simulink model "ctrl_PF"  (R2022b)
settings: Solver=FixedStepAuto  StartTime=0.0  StopTime=Tf  FixedStep=0.05  RelTol=1e-3
StopFcn:
  | save('testdata')
values from neighbouring files (symbols this model uses):
  Ba_0 = [0 0 0 0 0 0]    [run.m]    (also in testdata.mat)
  Bb = 4418825.3321    [testdata.mat]
  Bv_0 = [-5.14444 0 0 0 0 0]    [run.m]    (also in testdata.mat)
  Bx_0 = [-Cp(1,1) -Cp(2,1) Cp(3,1) 0 0 -pi]    [run.m]    (also in testdata.mat = [7.34788079488e-14 -400 -100 0 0 -3.14159265359])
  Cp = [x;y;z]    [run.m]    (also in testdata.mat = [-7.34788079488e-14 400 -100 -24.1026674607 399.273166418 -1)
  Cp_prime = Cp*Diff    [run.m]    (also in testdata.mat = [-4.77232815721 -0.143913049279 0 -4.75515990164 -0.42831409)
  d = 50    [run.m]    (also in testdata.mat)
  dA_BP1 = [0.00388591051125 0.00354364911083 0.00553040741788 0.00502167988714 0.0078585088908 0.00748424955325 0.0119232766011 0.0109054787122 0.0168329706434 0.016985509009 0.0156802934897 0.014556760782 ... (616 elements, 616x1)]    [testdata.mat]
  dA_BP2 = [0.00388594063171 0.00354357191533 0.00553040491113 0.00502170939051 0.00785855989083 0.00748435285791 0.0119232653011 0.0109054419481 0.0168329955973 0.0169854794658 0.015680230324 0.0145567225609 ... (616 elements, 616x1)]    [testdata.mat]
  dA_Hull = [0.896301676511 0.898896720864 0.884294141897 0.886832830172 0.870887902011 0.873360353662 0.856223658523 0.858613244346 0.840314828191 0.842595287849 0.823129385532 0.8253007603 ... (2914 elements, 2914x1)]    [testdata.mat]
  dA_PH = [0.00917454029683 0.00917454029683 0.00646521761836 0.00644666811643 0.011728531678 0.0107683420972 0.0165186720105 0.0100399866209 0.0121147162203 0.00917369783051 0.00917369783051 0.00646462373197 ... (550 elements, 550x1)]    [testdata.mat]
  dA_Sail = [0.08073747293 0.0655437895785 0.0678199581962 0.211496702297 0.185444652254 0.10949647106 0.0763960001413 0.0735864235671 0.0440728222699 0.281106392154 0.32735958292 0.104041938486 ... (564 elements, 564x1)]    [testdata.mat]
  dA_SProot = [0.0225345452169 0.0247277274893 0.0225345452169 0.0480467976325 0.0166447079844 0.0410754287554 0.0247277274893 0.0480467976325 0.0468898715351 0.0839833312794 0.0166447079844 0.0255016718 ... (904 elements, 904x1)]    [testdata.mat]
  dA_X1a = [0.0149621011817 0.0166706156701 0.0341149781095 0.0355915100668 0.0512235531199 0.0489176133683 0.0604458424392 0.0503279152264 0.0577124835488 0.0401555322121 0.044833653096 0.0251568218541 ... (200 elements, 200x1)]    [testdata.mat]
  dA_X1b = [0.0149621011817 0.0166706156701 0.0341149781095 0.0355915100668 0.0512235531199 0.0489176133683 0.0604458424392 0.0503279152264 0.0577124835488 0.0401555322121 0.044833653096 0.0251568218541 ... (200 elements, 200x1)]    [testdata.mat]
  dA_X2a = [0.0149620639393 0.0166705502855 0.0341150948266 0.0355913495849 0.051223110376 0.0489180393921 0.0604458270347 0.0503275686692 0.0577128112225 0.0401556683139 0.0448334591683 0.0251566482124 ... (200 elements, 200x1)]    [testdata.mat]
  dA_X2b = [0.0149620639393 0.0166705502855 0.0341150948266 0.0355913495849 0.051223110376 0.0489180393921 0.0604458270347 0.0503275686692 0.0577128112225 0.0401556683139 0.0448334591683 0.0251566482124 ... (200 elements, 200x1)]    [testdata.mat]
  dA_X3a = [0.0149621011817 0.0166706156701 0.0341149781095 0.0355915100668 0.0512235531199 0.0489176133683 0.0604458424392 0.0503279152264 0.0577124835488 0.0401555322121 0.044833653096 0.0251568218541 ... (200 elements, 200x1)]    [testdata.mat]
  dA_X3b = [0.0149621011817 0.0166706156701 0.0341149781095 0.0355915100668 0.0512235531199 0.0489176133683 0.0604458424392 0.0503279152264 0.0577124835488 0.0401555322121 0.044833653096 0.0251568218541 ... (200 elements, 200x1)]    [testdata.mat]
  dA_X4a = [0.0149621011817 0.0166706156701 0.0341149781095 0.0355915100668 0.0512235531199 0.0489176133683 0.0604458424392 0.0503279152264 0.0577124835488 0.0401555322121 0.044833653096 0.0251568218541 ... (200 elements, 200x1)]    [testdata.mat]
  dA_X4b = [0.0149621011817 0.0166706156701 0.0341149781095 0.0355915100668 0.0512235531199 0.0489176133683 0.0604458424392 0.0503279152264 0.0577124835488 0.0401555322121 0.044833653096 0.0251568218541 ... (200 elements, 200x1)]    [testdata.mat]
  Ixx = 52300000    [testdata.mat]
  Ixy = 0    [testdata.mat]
  Ixz = 0    [testdata.mat]
  Iyy = 1375000000    [testdata.mat]
  Iyz = 0    [testdata.mat]
  Izz = 1367000000    [testdata.mat]
  Ky = 1    [run.m]    (also in testdata.mat)
  Mb = 4418825.3321    [testdata.mat]
  n_BP1 = [-0.7747315 -0.03638153 -0.4095958 0 -0.1221389 0 -0.01670914 0 0.005209626 0 0.03404154 0 ... (1848 elements, 616x3)]    [testdata.mat]
  n_BP2 = [-0.774731517 -0.0363815315 -0.409595788 0 -0.122138903 0 -0.0167091396 0 0.00520962616 0 0.0340415388 0 ... (1848 elements, 616x3)]    [testdata.mat]
  n_Hull = [-3.334458e-05 -1.700098e-14 -3.354233e-05 -1.686235e-14 -3.289162e-05 -1.685701e-14 -3.291391e-05 -1.698144e-14 -3.338145e-05 -1.688959e-14 -3.29289e-05 -1.682536e-14 ... (8742 elements, 2914x3)]    [testdata.mat]
  n_PH = [0 0 0.01711651 0.01711627 0.2676807 0.2676804 0.7675173 0.7675174 0.9857236 0 0 0.01711456 ... (1650 elements, 550x3)]    [testdata.mat]
  n_Sail = [-0.05126832 -0.05168081 -0.0485872 -0.03288998 -0.03203588 -0.04435105 -0.04335441 -0.04419429 -0.05169604 0.01094904 0.01649325 -0.03825178 ... (1692 elements, 564x3)]    [testdata.mat]
  n_SProot = [-0.7837688 -0.7969784 -0.7837688 -0.79448 -0.280412 -0.3378876 -0.7969784 -0.79448 -0.7910827 -0.3483897 -0.280412 -0.2790298 ... (2712 elements, 904x3)]    [testdata.mat]
  n_X2a = [-0.283297986 -0.283136904 -0.283195704 -0.28313759 -0.2831586 -0.283137113 -0.28313911 -0.283136606 -0.283121586 -0.283136815 -0.283108413 -0.283138901 ... (600 elements, 200x3)]    [testdata.mat]
  n_X2b = [-0.283297986 -0.283136904 -0.283195704 -0.28313759 -0.2831586 -0.283137113 -0.28313911 -0.283136606 -0.283121586 -0.283136815 -0.283108413 -0.283138901 ... (600 elements, 200x3)]    [testdata.mat]
  n_X3a = [-0.283298 -0.2831369 -0.2831957 -0.2831376 -0.2831586 -0.2831371 -0.2831391 -0.2831366 -0.2831216 -0.2831368 -0.2831084 -0.2831389 ... (600 elements, 200x3)]    [testdata.mat]
  n_X4a = [-0.283298 -0.2831369 -0.2831957 -0.2831376 -0.2831586 -0.2831371 -0.2831391 -0.2831366 -0.2831216 -0.2831368 -0.2831084 -0.2831389 ... (600 elements, 200x3)]    [testdata.mat]
  n_X4b = [-0.283298 -0.2831369 -0.2831957 -0.2831376 -0.2831586 -0.2831371 -0.2831391 -0.2831366 -0.2831216 -0.2831368 -0.2831084 -0.2831389 ... (600 elements, 200x3)]    [testdata.mat]
  nt_BP1 = 616    [testdata.mat]
  nt_BP2 = 616    [testdata.mat]
  nt_Hull = 2914    [testdata.mat]
  nt_PH = 550    [testdata.mat]
  nt_Sail = 564    [testdata.mat]
  nt_SProot = 904    [testdata.mat]
  nt_X1a = 200    [testdata.mat]
  nt_X1b = 200    [testdata.mat]
  nt_X2a = 200    [testdata.mat]
  nt_X2b = 200    [testdata.mat]
  nt_X3a = 200    [testdata.mat]
  nt_X3b = 200    [testdata.mat]
  nt_X4a = 200    [testdata.mat]
  nt_X4b = 200    [testdata.mat]
  Seastate = 0    [run.m]    (also in testdata.mat)
  Tf = 500    [run.m]    (also in testdata.mat)
  v_ref = Bv_0(1)    [run.m]    (also in testdata.mat = -5.14444)
  vt1_BP1 = [-11.0524049722 -10.9924120522 -10.9924120522 -10.8819663922 -10.8819663922 -10.7297166322 -10.7297166322 -10.5070632922 -10.5070632922 -10.1807245522 -10.1807245522 -9.8815181122 ... (1848 elements, 616x3)]    [testdata.mat]
  vt1_BP2 = [-11.0524048318 -10.9924111396 -10.9924111396 -10.8819658306 -10.8819658306 -10.7297157898 -10.7297157898 -10.5070637134 -10.5070637134 -10.1807238502 -10.1807238502 -9.8815188844 ... (1848 elements, 616x3)]    [testdata.mat]
  vt1_Hull = [3.5122487678 3.7304022878 5.2621803278 5.4863499878 6.9866994878 7.2167238278 8.6832650078 8.9189474678 10.3493567078 10.5904445678 11.9823842078 12.2286247478 ... (8742 elements, 2914x3)]    [testdata.mat]
  vt1_PH = [37.3342788278 37.3342788278 37.4268866678 37.4268866678 37.5892452278 37.5892452278 37.7549453078 37.7549453078 37.8074619278 37.3342788278 37.3342788278 37.4268866678 ... (1650 elements, 550x3)]    [testdata.mat]
  vt1_Sail = [-12.4909433722 -12.1578443722 -12.0399645322 -11.2138368922 -10.6240515922 -11.5111900522 -11.9364967522 -11.6561249722 -12.4909433722 -7.5732648922 -6.8453119522 -11.1890071522 ... (1692 elements, 564x3)]    [testdata.mat]
  vt1_SProot = [29.2099766678 29.1371231078 29.0494854278 29.2099766678 29.2862630078 29.4526510478 29.0494854278 29.1261368078 29.3369263478 29.5706712878 29.0494854278 29.3857364078 ... (2712 elements, 904x3)]    [testdata.mat]
  vt1_X1a = [29.3961751478 29.4776282078 29.4776282078 29.7060309278 29.7060309278 30.0693861278 30.0693861278 30.5458756478 30.5458756478 31.0830460478 31.0830460478 31.6023926678 ... (600 elements, 200x3)]    [testdata.mat]
  vt1_X1b = [29.6638337078 29.6638337078 29.9620713878 29.9620713878 30.3181187678 30.3181187678 30.7116389078 30.7116389078 31.1104380878 31.1104380878 31.4810519678 31.4810519678 ... (600 elements, 200x3)]    [testdata.mat]
  vt1_X2a = [29.3961767624 29.4776272952 29.4776272952 29.7060326828 29.7060326828 30.0693842324 30.0693842324 30.5458736822 30.5458736822 31.083047171 31.083047171 31.6023916148 ... (600 elements, 200x3)]    [testdata.mat]
  vt1_X2b = [29.6638345502 29.6638345502 29.9620708964 29.9620708964 30.3181168022 30.3181168022 30.7116409436 30.7116409436 31.1104372454 31.1104372454 31.4810526698 31.4810526698 ... (600 elements, 200x3)]    [testdata.mat]
  vt1_X3a = [29.3961751478 29.4776282078 29.4776282078 29.7060309278 29.7060309278 30.0693861278 30.0693861278 30.5458756478 30.5458756478 31.0830460478 31.0830460478 31.6023926678 ... (600 elements, 200x3)]    [testdata.mat]
  vt1_X3b = [29.6638337078 29.6638337078 29.9620713878 29.9620713878 30.3181187678 30.3181187678 30.7116389078 30.7116389078 31.1104380878 31.1104380878 31.4810519678 31.4810519678 ... (600 elements, 200x3)]    [testdata.mat]
  vt1_X4a = [29.6638337078 29.6638337078 29.9620713878 29.9620713878 30.3181187678 30.3181187678 30.7116389078 30.7116389078 31.1104380878 31.1104380878 31.4810519678 31.4810519678 ... (600 elements, 200x3)]    [testdata.mat]
  vt1_X4b = [29.3961751478 29.4776282078 29.4776282078 29.7060309278 29.7060309278 30.0693861278 30.0693861278 30.5458756478 30.5458756478 31.0830460478 31.0830460478 31.6023926678 ... (600 elements, 200x3)]    [testdata.mat]
  vt2_BP1 = [-10.9924120522 -10.9494777322 -10.8819663922 -10.8505308322 -10.7297166322 -10.7112259522 -10.5070632922 -10.4997203722 -10.1807245522 -10.1757543922 -9.8815181122 -9.8813004922 ... (1848 elements, 616x3)]    [testdata.mat]
  vt2_BP2 = [-11.0294626294 -11.0294626294 -10.9494786448 -10.9494786448 -10.8505316746 -10.8505316746 -10.7112256012 -10.7112256012 -10.499720302 -10.499720302 -10.1757550942 -10.1757550942 ... (1848 elements, 616x3)]    [testdata.mat]
  vt2_Hull = [1.9517168078 1.9517168078 3.7304022878 3.7304022878 5.4863499878 5.4863499878 7.2167238278 7.2167238278 8.9189474678 8.9189474678 10.5904445678 10.5904445678 ... (8742 elements, 2914x3)]    [testdata.mat]
  vt2_PH = [37.2028433678 37.2028433678 37.3342788278 37.4268866678 37.4268866678 37.5892452278 37.5892452278 37.7549453078 37.7549453078 37.2028433678 37.2028433678 37.3342788278 ... (1650 elements, 550x3)]    [testdata.mat]
  vt2_Sail = [-12.0399645322 -12.0399645322 -11.9364967522 -10.7084881522 -10.7084881522 -12.0399645322 -12.0399645322 -11.9364967522 -12.3734566522 -7.7110323922 -7.7110323922 -11.6561249722 ... (1692 elements, 564x3)]    [testdata.mat]
  vt2_SProot = [29.0494854278 29.0494854278 29.2099766678 29.1261368078 29.0494854278 29.1371231078 29.1371231078 29.2099766678 29.1261368078 29.2099766678 29.2862630078 29.2862630078 ... (2712 elements, 904x3)]    [testdata.mat]
  vt2_X1a = [29.4776282078 29.9620713878 29.7060309278 30.3181187678 30.0693861278 30.7116389078 30.5458756478 31.1104380878 31.0830460478 31.4810519678 31.6023926678 31.7970362078 ... (600 elements, 200x3)]    [testdata.mat]
  vt2_X1b = [29.4776282078 29.9620713878 29.7060309278 30.3181187678 30.0693861278 30.7116389078 30.5458756478 31.1104380878 31.0830460478 31.4810519678 31.6023926678 31.7970362078 ... (600 elements, 200x3)]    [testdata.mat]
  vt2_X2a = [29.6638345502 29.6638345502 29.9620708964 29.9620708964 30.3181168022 30.3181168022 30.7116409436 30.7116409436 31.1104372454 31.1104372454 31.4810526698 31.4810526698 ... (600 elements, 200x3)]    [testdata.mat]
  vt2_X2b = [29.3961767624 29.4776272952 29.4776272952 29.7060326828 29.7060326828 30.0693842324 30.0693842324 30.5458736822 30.5458736822 31.083047171 31.083047171 31.6023916148 ... (600 elements, 200x3)]    [testdata.mat]
  vt2_X3a = [29.4776282078 29.9620713878 29.7060309278 30.3181187678 30.0693861278 30.7116389078 30.5458756478 31.1104380878 31.0830460478 31.4810519678 31.6023926678 31.7970362078 ... (600 elements, 200x3)]    [testdata.mat]
  vt2_X3b = [29.4776282078 29.9620713878 29.7060309278 30.3181187678 30.0693861278 30.7116389078 30.5458756478 31.1104380878 31.0830460478 31.4810519678 31.6023926678 31.7970362078 ... (600 elements, 200x3)]    [testdata.mat]
  vt2_X4a = [29.4776282078 29.9620713878 29.7060309278 30.3181187678 30.0693861278 30.7116389078 30.5458756478 31.1104380878 31.0830460478 31.4810519678 31.6023926678 31.7970362078 ... (600 elements, 200x3)]    [testdata.mat]
  vt2_X4b = [29.4776282078 29.9620713878 29.7060309278 30.3181187678 30.0693861278 30.7116389078 30.5458756478 31.1104380878 31.0830460478 31.4810519678 31.6023926678 31.7970362078 ... (600 elements, 200x3)]    [testdata.mat]
  vt3_BP1 = [-11.0294636122 -11.0294636122 -10.9494777322 -10.9494777322 -10.8505308322 -10.8505308322 -10.7112259522 -10.7112259522 -10.4997203722 -10.4997203722 -10.1757543922 -10.1757543922 ... (1848 elements, 616x3)]    [testdata.mat]
  vt3_BP2 = [-10.9924111396 -10.9494786448 -10.8819658306 -10.8505316746 -10.7297157898 -10.7112256012 -10.5070637134 -10.499720302 -10.1807238502 -10.1757550942 -9.8815188844 -9.8813013346 ... (1848 elements, 616x3)]    [testdata.mat]
  vt3_Hull = [1.7397198278 3.5122487678 3.5122487678 5.2621803278 5.2621803278 6.9866994878 6.9866994878 8.6832650078 8.6832650078 10.3493567078 10.3493567078 11.9823842078 ... (8742 elements, 2914x3)]    [testdata.mat]
  vt3_PH = [37.2028433678 37.3342788278 37.3342788278 37.3342788278 37.4268866678 37.4268866678 37.5892452278 37.5892452278 37.7549453078 37.2028433678 37.3342788278 37.3342788278 ... (1650 elements, 550x3)]    [testdata.mat]
  vt3_Sail = [-12.3734566522 -12.4909433722 -12.3734566522 -11.5111900522 -11.2138368922 -11.7698559922 -11.5111900522 -11.5111900522 -12.1578443722 -8.3109054322 -7.5732648922 -11.5111900522 ... (1692 elements, 564x3)]    [testdata.mat]
  vt3_SProot = [29.1261368078 29.2099766678 29.1261368078 29.3369263478 29.1371231078 29.2099766678 29.2099766678 29.3369263478 29.2548344678 29.3369263478 29.1371231078 29.1371231078 ... (2712 elements, 904x3)]    [testdata.mat]
  vt3_X1a = [29.6638337078 29.6638337078 29.9620713878 29.9620713878 30.3181187678 30.3181187678 30.7116389078 30.7116389078 31.1104380878 31.1104380878 31.4810519678 31.4810519678 ... (600 elements, 200x3)]    [testdata.mat]
  vt3_X1b = [29.3961751478 29.4776282078 29.4776282078 29.7060309278 29.7060309278 30.0693861278 30.0693861278 30.5458756478 30.5458756478 31.0830460478 31.0830460478 31.6023926678 ... (600 elements, 200x3)]    [testdata.mat]
  vt3_X2a = [29.4776272952 29.9620708964 29.7060326828 30.3181168022 30.0693842324 30.7116409436 30.5458736822 31.1104372454 31.083047171 31.4810526698 31.6023916148 31.7970343826 ... (600 elements, 200x3)]    [testdata.mat]
  vt3_X2b = [29.4776272952 29.9620708964 29.7060326828 30.3181168022 30.0693842324 30.7116409436 30.5458736822 31.1104372454 31.083047171 31.4810526698 31.6023916148 31.7970343826 ... (600 elements, 200x3)]    [testdata.mat]
  vt3_X3a = [29.6638337078 29.6638337078 29.9620713878 29.9620713878 30.3181187678 30.3181187678 30.7116389078 30.7116389078 31.1104380878 31.1104380878 31.4810519678 31.4810519678 ... (600 elements, 200x3)]    [testdata.mat]
  vt3_X3b = [29.3961751478 29.4776282078 29.4776282078 29.7060309278 29.7060309278 30.0693861278 30.0693861278 30.5458756478 30.5458756478 31.0830460478 31.0830460478 31.6023926678 ... (600 elements, 200x3)]    [testdata.mat]
  vt3_X4a = [29.3961751478 29.4776282078 29.4776282078 29.7060309278 29.7060309278 30.0693861278 30.0693861278 30.5458756478 30.5458756478 31.0830460478 31.0830460478 31.6023926678 ... (600 elements, 200x3)]    [testdata.mat]
  vt3_X4b = [29.6638337078 29.6638337078 29.9620713878 29.9620713878 30.3181187678 30.3181187678 30.7116389078 30.7116389078 31.1104380878 31.1104380878 31.4810519678 31.4810519678 ... (600 elements, 200x3)]    [testdata.mat]
  Xb = 0    [testdata.mat]
  Xcg = [32.3287332922 0 0]    [testdata.mat]
  Xg = 0    [testdata.mat]
  Yb = 0    [testdata.mat]
  Yg = 0    [testdata.mat]
  Zb = 0.4406    [testdata.mat]
  Zg = 0    [testdata.mat]
undefined symbols (not defined in the file or in its folder): Cpv
libraries: simulink x8, sharedtransform x2, dspmathops x2
(part 8 of 8)

== matlab function ctrl_PF/HDM/HDM B3/Wave, Virtual Mass and Hydrostatic/Wave Particle Motions/Sectional Wave Particle & Rigid Body Velocities ==
  data: time input; U_ship input; X_earth input; Xce input size=[15 3]; Rs input size=[15 3]; phi_wave input; beta_wave input; Uws output size=[15 3]; L_wave input; A_wave input; k_wave input; w_wave input; Urs output size=[15 3]
function [Uws,Urs] = fcn(time,U_ship,X_earth,Xce,Rs,phi_wave,beta_wave,L_wave,A_wave,k_wave,w_wave)
%Inputs
%Rs      : Position vector of each sectional component in ship system.
%X_earth : Global ship position in the earth coordinate system
%U_ship  : Ship's velocity at CG in the ship coordinate system
%L, A, T, k, w of wave: wave properties for given sea state

%Outputs
%Uws: Sectional wave particle velcity vector in ship coordinate system
%Urs: Sectional rigid body translationl velocity vector in ship coordinate system

phi= X_earth(4); theta= X_earth(5); psi= X_earth(6); % Euler angles
u_s= U_ship(1); v_s=U_ship(2); w_s=U_ship(3); p_s= U_ship(4); q_s=U_ship(5); r_s=U_ship(6);

ni = 15; %length(Xce); %number, and the order of sectional elements

Uws = zeros(15,3); Urs = zeros(15,3);
uweBow=zeros(3,1); uweStern=zeros(3,1); uweBP=zeros(3,1);
ursProbe=zeros(3,1);

uri=zeros(15,1); vri=zeros(15,1); wri=zeros(15,1);
uwi=zeros(15,1); vwi=zeros(15); wwi=zeros(15,1);

Omega_s = [p_s; q_s; r_s;]; %angular velocity of the CG in ship coordinate system
Us_CG   = [u_s; v_s; w_s;]; %Translational velocity of the CG in ship coordinate system

RMat=[cos(theta)*cos(psi) -cos(phi)*sin(psi)+sin(phi)*sin(theta)*cos(psi)  sin(phi)*sin(psi)+cos(phi)*sin(theta)*cos(psi); ...
      cos(theta)*sin(psi)  cos(phi)*cos(psi)+sin(phi)*sin(theta)*sin(psi) -sin(phi)*cos(psi)+cos(phi)*sin(theta)*sin(psi); ...
     -sin(theta)                             sin(phi)*cos(theta)                             cos(phi)*cos(theta)];

%phi_wave  = 0; % wave phase. parameterized
%beta_wave = 0; % wave heading. parameterized

    for i= 1:15
        u_w=-A_wave*w_wave*exp(k_wave*Xce(i,3))*cos(k_wave*Xce(i,1)-w_wave*time+phi_wave)*cos(pi*beta_wave);
        v_w= A_wave*w_wave*exp(k_wave*Xce(i,3))*cos(k_wave*Xce(i,1)-w_wave*time+phi_wave)*sin(pi*beta_wave);
        w_w=-A_wave*w_wave*exp(k_wave*Xce(i,3))*sin(k_wave*Xce(i,1)-w_wave*time+phi_wave);
        
        v1=u_w; v2=v_w; v3=w_w;
        uwi(i,1)=v1; vwi(i,1)=v2; wwi(i,1)=v3;
        
        Uwe = [u_w; v_w; w_w;];
        Uint= inv(RMat)*Uwe;
        Uws(i,:) = Uint(:);  %keep Uws for further use in wave AOA calculation     

        if i==1
            uweBow=Uwe;
        elseif i==10
            uweStern=Uwe;
        elseif i==14
            uweBP=Uwe;
        end
        
    end
    
    %Computation of translational velcity of volumetric center of sections.   
    for i=1:15
        r_i      = [Rs(i,1); Rs(i,2); Rs(i,3)];
        Ur_int   = Us_CG + cross(Omega_s,r_i); %cross(r_i,Omega_s);
        
        v1=Ur_int(1); v2=Ur_int(2); v3=Ur_int(3); 
        uri(i,1)=v1; vri(i,1)=v2; wri(i,1)=v3;
        
        for j=1:3
            Urs(i,j)=Ur_int(j);    
        end
    end

end

== matlab function ctrl_PF/HDM/HDM B3/Wave, Virtual Mass and Hydrostatic/Wave Particle Motions/Wave Properties ==
  data: SeaState input; L_wave output; A_wave output; k_wave output; w_wave output
function [L_wave,A_wave,k_wave,w_wave] = fcn(SeaState)

   if SeaState==2;
       L_wave= 87.8; A_wave= 0.15;
   elseif SeaState==3;
       L_wave= 87.8; A_wave= 0.44;
   elseif SeaState==4;
       L_wave= 120.9; A_wave= 0.94;
   elseif SeaState==5;
       L_wave= 140.9; A_wave= 1.625;
   elseif SeaState==6;
       L_wave=240.1; A_wave=2.5;
   elseif SeaState==7;
       L_wave= 351.3; A_wave= 3.750;
   else
       L_wave= 0; A_wave=0;
   end
   
   if(L_wave==0)
       k_wave=0;
   else
       k_wave=2*pi/L_wave;
   end
   
   w_wave=sqrt(9.81*k_wave);
   
end

== matlab function ctrl_PF/HDM/HDM B3/Wave, Virtual Mass and Hydrostatic/Wave Particle Motions/Wave particle velocity at hull CG ==
  data: time input; X_earth input; uwsCG output; dLCG input; L_wave input; phi_wave input; beta_wave input; A_wave input; k_wave input; w_wave input
function uwsCG  = fcn(time,X_earth,dLCG,L_wave,phi_wave,beta_wave,A_wave,k_wave,w_wave)
 
    Xs=[X_earth(1); X_earth(2); X_earth(3);];
    phi= X_earth(4); theta= X_earth(5); psi= X_earth(6); % Euler angles
    
    RMat=[cos(theta)*cos(psi) -cos(phi)*sin(psi)+sin(phi)*sin(theta)*cos(psi)  sin(phi)*sin(psi)+cos(phi)*sin(theta)*cos(psi); ...
          cos(theta)*sin(psi)  cos(phi)*cos(psi)+sin(phi)*sin(theta)*sin(psi) -sin(phi)*cos(psi)+cos(phi)*sin(theta)*sin(psi); ...
        -sin(theta)                             sin(phi)*cos(theta)                             cos(phi)*cos(theta)];  

    u_w=-A_wave*w_wave*exp(k_wave*Xs(3))*cos(k_wave*Xs(1)-w_wave*time+phi_wave)*cos(pi*beta_wave);
    v_w= A_wave*w_wave*exp(k_wave*Xs(3))*cos(k_wave*Xs(1)-w_wave*time+phi_wave)*sin(pi*beta_wave);
    w_w=-A_wave*w_wave*exp(k_wave*Xs(3))*sin(k_wave*Xs(1)-w_wave*time+phi_wave);
    
    uweCG = [u_w; v_w; w_w;];
    uwsCG = inv(RMat)*uweCG;
    
end

== matlab function ctrl_PF/HDM/HDM B3/Wave, Virtual Mass and Hydrostatic/Wave Particle Motions/Wave particle velocity at the center of Appendages ==
  data: time input; rX1 input; uwX1s output; rX2 input; uwX2s output; uwX3s output; uwX4s output; uwXBs output; rX3 input; rX4 input; rXB input; X_earth input; U_ship input; L_wave input; phi_wave input; beta_wave input; A_wave input; k_wave input; w_wave input
function [uwX1s,uwX2s,uwX3s,uwX4s,uwXBs]= fcn(time,rX1,rX2,rX3,rX4,rXB,X_earth,U_ship,L_wave,phi_wave,beta_wave,A_wave,k_wave,w_wave)

    %rXi: position vector of Stern planes from the CG
    %rXB: position vector of sail planes from the CG
    %U_ship: rigid body velcity in the ship system

    phi= X_earth(4); theta= X_earth(5); psi= X_earth(6); % Euler angles
    %u_s= U_ship(1); v_s=U_ship(2); w_s=U_ship(3); p_s= U_ship(4); q_s=U_ship(5); r_s=U_ship(6);

    RMat=[cos(theta)*cos(psi) -cos(phi)*sin(psi)+sin(phi)*sin(theta)*cos(psi)  sin(phi)*sin(psi)+cos(phi)*sin(theta)*cos(psi); ...
          cos(theta)*sin(psi)  cos(phi)*cos(psi)+sin(phi)*sin(theta)*sin(psi) -sin(phi)*cos(psi)+cos(phi)*sin(theta)*sin(psi); ...
        -sin(theta)                             sin(phi)*cos(theta)                             cos(phi)*cos(theta)];

    Xhe=[X_earth(1); X_earth(2); X_earth(3);];
 
    X1e=Xhe+RMat*rX1;
    X2e=Xhe+RMat*rX2;
    X3e=Xhe+RMat*rX3;
    X4e=Xhe+RMat*rX4;
    XBe=Xhe+RMat*rXB;
 
    u_w=-A_wave*w_wave*exp(k_wave*X1e(3))*cos(k_wave*X1e(1)-w_wave*time+phi_wave)*cos(pi*beta_wave);
    v_w= A_wave*w_wave*exp(k_wave*X1e(3))*cos(k_wave*X1e(1)-w_wave*time+phi_wave)*sin(pi*beta_wave);
    w_w=-A_wave*w_wave*exp(k_wave*X1e(3))*sin(k_wave*X1e(1)-w_wave*time+phi_wave);
    uwX1e=[u_w; v_w; w_w;];
    
    u_w=-A_wave*w_wave*exp(k_wave*X2e(3))*cos(k_wave*X2e(1)-w_wave*time+phi_wave)*cos(pi*beta_wave);
    v_w= A_wave*w_wave*exp(k_wave*X2e(3))*cos(k_wave*X2e(1)-w_wave*time+phi_wave)*sin(pi*beta_wave);
    w_w=-A_wave*w_wave*exp(k_wave*X2e(3))*sin(k_wave*X2e(1)-w_wave*time+phi_wave);
    uwX2e=[u_w; v_w; w_w;];
 
    u_w=-A_wave*w_wave*exp(k_wave*X3e(3))*cos(k_wave*X3e(1)-w_wave*time+phi_wave)*cos(pi*beta_wave);
    v_w= A_wave*w_wave*exp(k_wave*X3e(3))*cos(k_wave*X3e(1)-w_wave*time+phi_wave)*sin(pi*beta_wave);
    w_w=-A_wave*w_wave*exp(k_wave*X3e(3))*sin(k_wave*X3e(1)-w_wave*time+phi_wave);
    uwX3e=[u_w; v_w; w_w;];
    
    u_w=-A_wave*w_wave*exp(k_wave*X4e(3))*cos(k_wave*X4e(1)-w_wave*time+phi_wave)*cos(pi*beta_wave);
    v_w= A_wave*w_wave*exp(k_wave*X4e(3))*cos(k_wave*X4e(1)-w_wave*time+phi_wave)*sin(pi*beta_wave);
    w_w=-A_wave*w_wave*exp(k_wave*X4e(3))*sin(k_wave*X4e(1)-w_wave*time+phi_wave);
    uwX4e=[u_w; v_w; w_w;];
    
    u_w=-A_wave*w_wave*exp(k_wave*XBe(3))*cos(k_wave*XBe(1)-w_wave*time+phi_wave)*cos(pi*beta_wave);
    v_w= A_wave*w_wave*exp(k_wave*XBe(3))*cos(k_wave*XBe(1)-w_wave*time+phi_wave)*sin(pi*beta_wave);
    w_w=-A_wave*w_wave*exp(k_wave*XBe(3))*sin(k_wave*XBe(1)-w_wave*time+phi_wave);
    uwXBe=[u_w; v_w; w_w;];
    
    uwX1s=inv(RMat)*uwX1e;
    uwX2s=inv(RMat)*uwX2e;
    uwX3s=inv(RMat)*uwX3e;
    uwX4s=inv(RMat)*uwX4e;
    uwXBs=inv(RMat)*uwXBe;
    
end

== matlab function ctrl_PF/HDM/HDM B3/X/Fx ==
  data: Bx input; Bv input; Ba input; CXqq input; CXuvwV input; CXuvwH input; Umag input; dLCG input; dmass input; UeSP input; XdXi input; X output; Tprop input; Mb parameter; Bb parameter; Xvm input; Xapp output; Xhull output; Tout output; X_Hyd output; XdX output; BFX input; Xstat output
function [X,Xapp,Xhull,Tout,X_Hyd,XdX,Xstat]   = fcn(Bx,Bv,Ba,CXqq,CXuvwV,CXuvwH,Umag,dLCG,dmass,UeSP,XdXi,Tprop,Mb,Bb,Xvm,BFX)
%Bx,Bv,Ba are the body motion position, velocity, acceleration in ship coordinate
%Wv,Wa are the wave particle velocity, acceleration in ship coordinate

u=Bv(1); v=Bv(2); w=Bv(3); p=Bv(4); q=Bv(5); r=Bv(6);
x=Bx(1); y=Bx(2); z=Bx(3); phi=Bx(4); theta=Bx(5); psi=Bx(6);
a1=Ba(1); a2=Ba(2); a3=Ba(3); a4=Ba(4); a5=Ba(5); a6=Ba(6); 

%Xwq=1025*70.2^3*CXwq
%Twq=0.5*1025*70.2^3*CTwq
%Xstat=BFX-(Mb+dmass)*9.81*sin(Bx(5));%-((Mb+dmass)-Bb)*9.81*sin(Bx(5));

Xqq=0.5*1025*70.2^4*q^2*CXqq;
Xwq=1025*70.2^3*(-3.3124286E-03*w*q)
Xvr=1025*70.2^3*(-3.3124286E-03*v*r)*0
Twq=0.5*1025*70.2^3*(3.6594E-03*w*q)
Tvr=0.5*1025*70.2^3*(3.6594E-03*v*r)*0

dXiuq=(4.4603E-03*(u*q)^2-7.3687E-06*(u*q))


XX1=0.5*1025*70.2^2*(XdXi(1)+dXiuq)*UeSP(1)^2
XX2=0.5*1025*70.2^2*(XdXi(2)+dXiuq)*UeSP(2)^2
XX3=0.5*1025*70.2^2*(XdXi(3)+dXiuq)*UeSP(3)^2
XX4=0.5*1025*70.2^2*(XdXi(4)+dXiuq)*UeSP(4)^2
XXB=0.5*1025*(70.2^2*XdXi(5)*UeSP(5)^2)

XdX=[XX1; XX2; XX3; XX4; XXB;]

Xapp=XX1+XX2+XX3+XX4+XXB;
Xuvw=-0.5*1025*70.2^2*(CXuvwV+CXuvwH)*Umag^2*u/abs(u);
Xstat=BFX+(Mb+dmass)*9.81*sin(Bx(5))
Xhull=Xqq+Xuvw+Xwq+Xvr;
Tout=Tprop+Twq+Tvr;
X_Hyd=Xapp+Xhull+Xstat-Tout;
X=Xapp+Xhull+Xstat-Tout+Xvm;

== matlab function ctrl_PF/HDM/HDM B3/Y/Fy ==
  data: Bx input; Bv input; Ba input; CYr input; CYvr input; CYrr input; CYuvw input; Umag input; UeX input; dLCG input; dmass input; CYdXi input; Mb parameter; Bb parameter; Fy output; FYApp output; FYhull output; FY_hyd output; FYprop output; Yvm input; FYAppAll output; BFY input; FYHullVM output
 function [Fy,FYApp,FYhull,FY_hyd,FYprop,FYAppAll,FYHullVM]  = fcn(Bx,Bv,Ba,CYr,CYvr,CYrr,CYuvw,Umag,UeX,dLCG,dmass,CYdXi,Mb,Bb,Yvm,BFY)
%Bx,Bv,Ba are the body motion position, velocity, acceleration in ship coordinate
%Wv,Wa are the wave particle velocity, acceleration in ship coordinate
 
u=Bv(1); v=Bv(2); w=Bv(3); p=Bv(4); q=Bv(5); r=Bv(6);
x=Bx(1); y=Bx(2); z=Bx(3); phi=Bx(4); theta=Bx(5); psi=Bx(6);
a1=Ba(1); a2=Ba(2); a3=Ba(3); a4=Ba(4); a5=Ba(5); a6=Ba(6); 

FYuvw=0.5*1025*70.2^2*CYuvw*Umag^2

FYx1=1025*70.2^2*CYdXi(1)*UeX(1)^2
FYx2=1025*70.2^2*CYdXi(2)*UeX(2)^2
FYx3=1025*70.2^2*CYdXi(3)*UeX(3)^2
FYx4=1025*70.2^2*CYdXi(4)*UeX(4)^2

FYrr=0.5*1025*70.2^4*CYrr*q*abs(q)*0
FYr =-1025*70.2^2*(0.9*8.2086E-03*u*r)*u^2*2

FYAppAll=[FYx1; FYx2 ;FYx3; FYx4;]

%FYr =0.5*1025*70.2^3*CYr*u^2*2
FYvr=0.5*1025*70.2^3*CYvr*u^2*0
FYprop=0;
FYhull=FYuvw+FYr+FYvr+FYrr
FYHullVM=FYhull+Yvm
FYApp=FYx1+FYx2+FYx3+FYx4
FYStat=(Mb+dmass)*9.81*cos(theta)*sin(phi)-BFY %((Mb+dmass)-Bb)*9.81*cos(theta)*sin(phi)
FY_hyd=FYApp+FYStat+FYhull+FYprop
Fy=FYApp+FYStat+FYhull+Yvm+FYprop
 end

== matlab function ctrl_PF/HDM/HDM B3/Z/Fz ==
  data: Bx input; Bv input; Ba input; Zqq input; Zuq input; Zwq input; Zuvw_a input; Zuvw_b input; CZProp input; Umag input; UeSP input; dLCG input; dmass input; ZdXi input; Mb parameter; Bb parameter; Fz output; Zvm input; FZApp output; FZHull output; FZProp output; FZ_Hyd output; FZApp_All output; BFZ input
 function [Fz,FZApp,FZHull,FZProp,FZ_Hyd,FZApp_All]  = fcn(Bx,Bv,Ba,Zqq,Zuq,Zwq,Zuvw_a,Zuvw_b,CZProp,Umag,UeSP,dLCG,dmass,ZdXi,Mb,Bb,Zvm,BFZ)
%Bx,Bv,Ba are the body motion position, velocity, acceleration in ship coordinate
%Wv,Wa are the wave particle velocity, acceleration in ship coordinate
 
u=Bv(1); v=Bv(2); w=Bv(3); p=Bv(4); q=Bv(5); r=Bv(6);
x=Bx(1); y=Bx(2); z=Bx(3); phi=Bx(4); theta=Bx(5); psi=Bx(6);
a1=Ba(1); a2=Ba(2); a3=Ba(3); a4=Ba(4); a5=Ba(5); a6=Ba(6); 

FZProp=0.5*1025*70.2^3*CZProp;

FZx1=0.5*1025*70.2^2*ZdXi(1)*UeSP(1)^2;
FZx2=0.5*1025*70.2^2*ZdXi(2)*UeSP(2)^2;
FZx3=0.5*1025*70.2^2*ZdXi(3)*UeSP(3)^2;
FZx4=0.5*1025*70.2^2*ZdXi(4)*UeSP(4)^2;
FZxb=0.5*1025*70.2^2*ZdXi(5)*UeSP(5)^2;

FZqq=0.5*1025*70.2^4*Zqq*q^2*5.1444^2;
FZuq=(-0.01066*u*q)*0.5*70.2^3*1025*0.6;
FZur=(1.5483E-03*u*r)*70.2^2*1025*5.1444^2;
FZwq=0.5*1025*70.2^3*Zwq*w*abs(q);

FZApp_All=[FZx1; FZx2; FZx3; FZx4; FZxb;];

FZApp=(FZx1+FZx2+FZx3+FZx4+FZxb);
FZuvw=0.5*1025*70.2^2*(Zuvw_a+Zuvw_b*2)*Umag^2;
FZStat=BFZ-((Mb+dmass))*9.81*cos(theta);
FZHull=FZuvw+FZqq+FZuq+FZur;
FZ_Hyd=FZApp+FZStat+FZHull+FZProp;

Fz=FZApp+FZStat+FZHull+FZProp+Zvm;
end

== matlab function ctrl_PF/HDM/HDM B3/Z/Linearized Zuvw ==
  data: x input; y output
function y = fcn(x)
y=2.5079E-04*1*x + 1.9855E-05
end

== matlab function ctrl_PF/HDM/Integration and Coord. Transfrom/Coordinate Transform/MATLAB Function2 ==
  data: Bx input; out output; Bv input
function out = fcn(Bx,Bv)
u = Bv(1); v = Bv(2); w = Bv(3); p = Bv(4); q = Bv(5); r = Bv(6);
x = Bx(1); y = Bx(2); z = Bx(3); phi = Bx(4); theta = Bx(5); psi = Bx(6);

Vx_ship=[u; v; w];
Vr_ship=[p; q; r];

RMat=[cos(theta)*cos(psi) -cos(phi)*sin(psi)+sin(phi)*sin(theta)*cos(psi)  sin(phi)*sin(psi)+cos(phi)*sin(theta)*cos(psi); ...
      cos(theta)*sin(psi)  cos(phi)*cos(psi)+sin(phi)*sin(theta)*sin(psi) -sin(phi)*cos(psi)+cos(phi)*sin(theta)*sin(psi); ...
              -sin(theta)                             sin(phi)*cos(theta)                             cos(phi)*cos(theta)];

QMat=[1  tan(theta)*sin(phi) tan(theta)*cos(phi); ...
      0  cos(phi)           -sin(phi); ...
      0  sin(phi)/cos(theta) cos(phi)/cos(theta)];
   
Vx_earth=RMat*Vx_ship;
Vr_earth=QMat*Vr_ship;


out = [Vx_earth(1); Vx_earth(2); Vx_earth(3); Vr_earth(1); Vr_earth(2); Vr_earth(3)];

== matlab function ctrl_PF/HDM/Integration and Coord. Transfrom/Rigid Body Motion/MATLAB Function2 ==
  data: X input; Y input; Z input; K input; M input; N input; out output; bx input; bv input; Mb parameter; Xg parameter; Zg parameter; Iyy parameter; Yg parameter; Yb parameter; Zb parameter; Ixx parameter; Izz parameter; Ixy parameter; Ixz parameter; Iyz parameter; Bb parameter; Xb parameter
function out = fcn(X,Y,Z,K,M,N,bx,bv,Mb,Xg,Zg,Iyy,Yg,Yb,Zb,Ixx,Izz,Ixy,Ixz,Iyz,Bb,Xb)

x = bx(1); y = bx(2); z = bx(3); phi = bx(4); theta = bx(5); psi = bx(6);
u = bv(1); v = bv(2); w = bv(3); p = bv(4);   q = bv(5);     r = bv(6);
F = [X; Y; Z; K; M; N];

A= [Mb 0 0 0 Mb*Zg -Mb*Yg; ...
     0 Mb 0 -Mb*Zg 0 Mb*Xg; ...
     0 0 Mb Mb*Yg -Mb*Xg 0; ...
     0 -Mb*Zg Mb*Yg Ixx -Ixy -Ixz; ...
     Mb*Zg 0 -Mb*Xg -Ixy Iyy -Iyz; ...
     -Mb*Yg Mb*Zg 0 -Ixz -Iyz Izz];
    
B= [Mb*(w*q-v*r-Xg*(q^2+r^2)+Yg*p*q+Zg*p*r); ...
     Mb*(u*r-w*p-Yg*(r^2+p^2)+Zg*q*r+Xg*p*q); ...
     Mb*(v*p-u*q-Zg*(p^2+q^2)+Xg*r*p+Yg*r*q); ...
    (Ixx-Iyy)*q*r+Mb*(Yg*(v*p-u*q)-Zg*(u*r-w*p)); ...
    (Ixx-Izz)*r*p+Mb*(Zg*(w*q-v*r)-Xg*(v*p-u*q)); ...
    (Iyy-Ixx)*p*q+Mb*(Xg*(u*r-w*p)-Yg*(w*q-v*r))];

%B = [Mb -Mb*Xg 0; 0 -Mb*Zg -Mb; Mb*Zg 0 Mb*Xg];

out = inv(A)*(F-B);

%out = [out_temp(1) ; out_temp(2) ; out_temp(3) ; out_temp(4) ; out_temp(5) ; out_temp(6)];

end
